simulink model "tester22"  (R2022b)
settings: Solver=VariableStepAuto  StartTime=0.0  StopTime=10  RelTol=1e-3
values from neighbouring files (symbols this model uses):
  Bf = [0.00436 0.00065 0.0119210 0.0127548 0.007765]*10000    [dane.m]    (also in tester23.m = [0.00436 0.00065 1.19210 1.27548 0.007765]; wykresownik33.m = [0.00436 0.00065 1.19210 1.27548 0.007765]; wykresownik35.m = [0.00436 0.00065 1.19210 1.27548 0.007765]; wykresownik36.m = [0.00436 0.00065 1.19210 1.27548 0.007765])
settings Model: Creator=48519  LastModifiedBy=48519
settings ModelReferenceCC: EnableRefExpFcnMdlSchedulingChecks=on

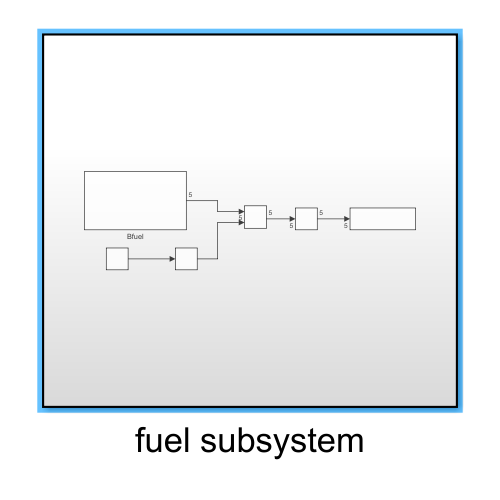
[thumbnail: Simulink's stored preview of the top-level diagram]
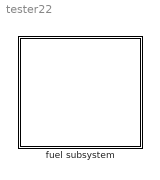
== system tester22 ==
  fuel subsystem : Subsystem

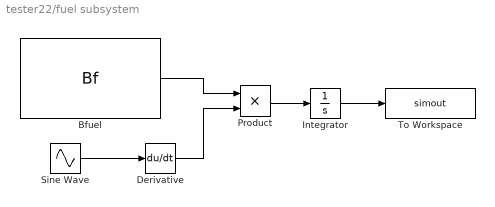
== system tester22/fuel subsystem ==
  Bfuel : Constant  Value=Bf
  Derivative : Derivative
  Integrator : Integrator  InitialCondition=1
  Product : Product
  Sine Wave : Sin  Amplitude=10  SampleTime=0.001
  To Workspace : ToWorkspace  VariableName=simout  SaveFormat=Timeseries  SampleTime=-1
  wires:
  Bfuel/1 -> Product/1
  Sine Wave/1 -> Derivative/1
  Derivative/1 -> Product/2
  Product/1 -> Integrator/1
  Integrator/1 -> To Workspace/1
